simulink model "DCDC_SEPIC_TopLevelModel"  (R2023b)
settings: Solver=ode23t  StartTime=0.0  StopTime=10  FixedStep=ts500us  RelTol=1e-3
StartFcn:
  | try
  | resetTiLeds(objLEDs);
  | end
undefined symbols (not defined in the file): GPTRIP1SEL, GPTRIP2SEL, operatingMode, psu_V, timer_period_LED, timer_period_SEPIC, ts, ts100ms, ts10ms, ts1ms, ts500us, TZ1, TZ2
libraries: fl_lib x34, ee_lib x18, dspstat3 x17, SEPIC_utilities x16, c2802xlib x13, nesl_utility x10, simulink x4, batteryecm_lib x3
(part 1 of 2)
CloseFcn:
  | clear objLEDs; close all force; clc;
settings Model: ExtModeTrigDuration=8  Creator=vivekr  LastModifiedBy=vlenzi
settings SolverCC: AlgebraicLoopSolver=TrustRegion
settings DataIOCC: SaveFormat=StructureWithTime  SaveOutput=off  SaveTime=off  SignalLoggingName=logsOut
settings OptimizationCC: DefaultParameterBehavior=Inlined  UseDivisionForNetSlopeComputation=UseDivisionForReciprocalsOfIntegersOnly  EnhancedBackFolding=on  BooleansAsBitfields=on  PassReuseOutputArgsAs=Individual arguments  ExpressionDepthLimit=2147483647  StateBitsets=on  DataBitsets=on  ZeroExternalMemoryAtStartup=off  NoFixptDivByZeroProtection=on  EfficientFloat2IntCast=on  LifeSpan=1  MaxStackSize=64  SimCompilerOptimization=on  EfficientTunableParamExpr=on
settings DebuggingCC: ReadBeforeWriteMsg=DisableAll  WriteAfterWriteMsg=DisableAll  WriteAfterReadMsg=DisableAll  UnderspecifiedInitializationDetection=Classic  CheckExecutionContextPreStartOutputMsg=on  ParameterPrecisionLossMsg=none  FcnCallInpInsideContextMsg=warning  UnconnectedInputMsg=warning  UnconnectedOutputMsg=warning  UnconnectedLineMsg=warning  UniqueDataStoreMsg=error  AllowSymbolicDim=off  ModelReferenceSymbolNameMessage=none  StateNameClashWarn=warning  StrictBusMsg=ErrorOnBusTreatedAsVector  SymbolicDimsDataTypeCodeGenerationDiagnostic=none  SFUnexpectedBacktrackingDiag=warning  SFNoUnconditionalDefaultTransitionDiag=warning  SFExecutionAtInitializationDiag=none  ArithmeticOperatorsInVariantConditions=warning
settings HardwareCC: TargetHWDeviceType=Generic->32-bit Embedded Processor
settings ModelReferenceCC: EnableRefExpFcnMdlSchedulingChecks=on  CheckModelReferenceTargetMessage=none  PropagateSignalLabelsOutOfModel=off
settings SFSimCC: SimUseLocalCustomCode=off  MATLABDynamicMemAlloc=off
settings RTWCC: Description=Embedded Coder  SystemTargetFile=ert.tlc  TemplateMakefile=ert_default_tmf  GenerateReport=on  RTWVerbose=off  RTWUseLocalCustomCode=off  Toolchain=Texas Instruments Code Composer Studio (C2000)  IncludeHyperlinkInReport=on  CodeExecutionProfiling=on  CodeProfilingSaveOptions=AllData  CodeProfilingInstrumentation=coarse  GenerateTraceInfo=on  GenerateTraceReport=on  GenerateTraceReportSl=on  GenerateTraceReportSf=on  GenerateTraceReportEml=on  GenerateCodeMetricsReport=on  DLArmComputeVersion=19.05
settings CodeAppCC: ForceParamTrailComments=on  IgnoreCustomStorageClasses=off  SimulinkDataObjDesc=on  CustomSymbolStrGlobalVar=rt$N$M  CustomSymbolStrType=$N$M  CustomSymbolStrFcn=$N$M$F  CustomSymbolStrMacro=$N$M  InsertBlockDesc=on  StateflowObjectComments=on  InternalIdentifier=Classic
settings ERTTargetCC: UtilityFuncGeneration=Shared location  MultiwordLength=2048  IncludeMdlTerminateFcn=off  CombineSignalStateStructs=on  SupportNonFinite=off  SupportComplex=off  ExtModeStaticAllocSize=2048  ERTCustomFileTemplate=example_file_process.tlc  ERTFilePackagingFormat=CompactWithDataFile  ConvertIfToSwitch=off  SuppressUnreachableDefaultCases=off
settings ConfigComp: CovMetricSettings=dw  CovSaveCumulativeToWorkspaceVar=on  CovSaveSingleToWorkspaceVar=on  CovExternalEMLEnable=off  CovSFcnEnable=off
settings SimscapeCC: SimscapeUseOperatingPoints=on  SimscapeOperatingPoint=op_tm_average

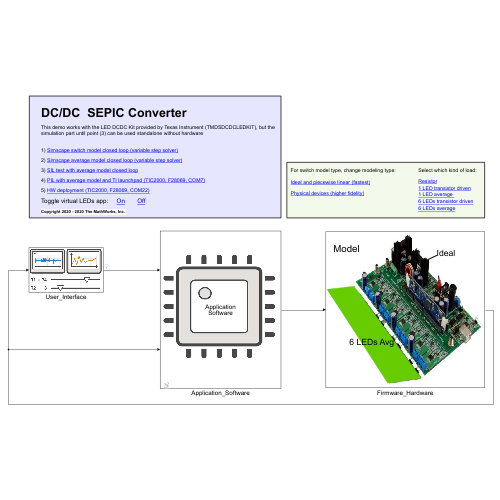
[thumbnail: Simulink's stored preview of the top-level diagram]
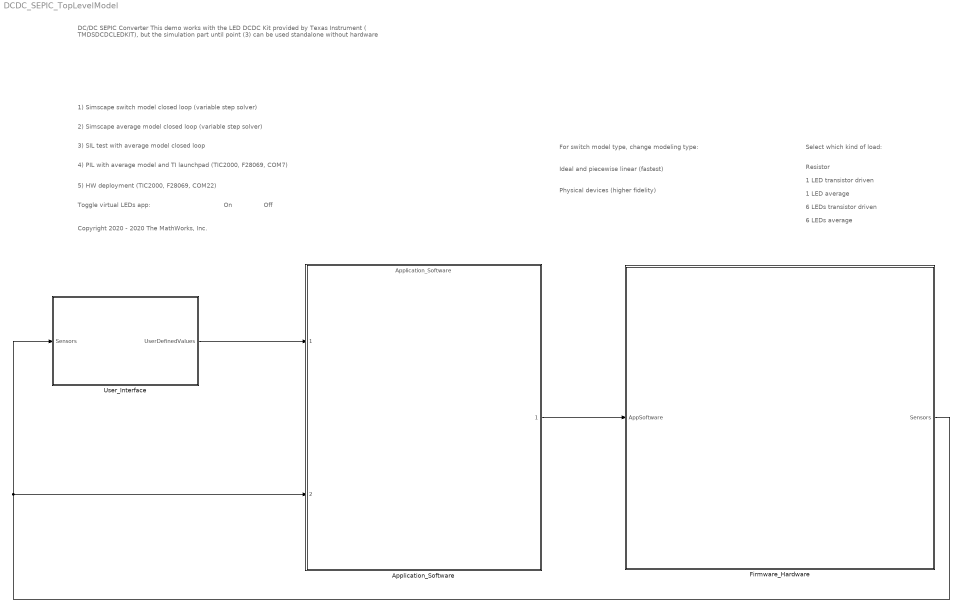
== system DCDC_SEPIC_TopLevelModel ==
  note: Copyright 2020 - 2020 The MathWorks, Inc.
  note: Ideal and piecewise linear (fastest)
  note: DC/DC SEPIC Converter
      |
      | This demo works with the LED DCDC Kit provided by Texas Instrument ( TMDSDCDCLEDKIT), but the simulation part until point (3) can be used standalone without hardware
  note: 5) HW deployment (TIC2000, F28069, COM22)
  note: 2) Simscape average model closed loop (variable step solver)
  note: 1) Simscape switch model closed loop (variable step solver)
  note: Physical devices (higher fidelity)
  note: For switch model type, change modeling type:
  note: 3) SIL test with average model closed loop
  note: Select which kind of load:
  note: Resistor
  note: 1 LED transistor driven
  note: 1 LED average
  note: 6 LEDs transistor driven
  note: 6 LEDs average
  note: Toggle virtual LEDs app:
  note: On
  note: Off
  note: 4) PIL with average model and TI launchpad (TIC2000, F28069, COM7)
  Application_Software : ModelReference  ModelNameDialog=Application_Software  SimulationMode=Normal  ModelReferenceVersion=1.589
      mask Display: image('cpu.png');disp('Application\nSoftware');
  Firmware_Hardware : Subsystem
      mask Display: image('SEPIC_converter_TI_Kit.jpg');text(0.05,0.9,'\fontsize{28}Model','texmode', 'on');plot([0.6 0.7],[0.8 0.85]);text(0.7,0.87,'\fontsize{25}Ideal','texmode', 'on');patch([0.39 0.01 0.18 0.6],[0.03 0.63 0.65 0.06], [0.4 0.8 0]);text(0.15,0.3,'\fontsize{25}6 LEDs Avg','texmode', 'on');
  User_Interface : Subsystem
      mask Display: image('user_interface.png');
  wires:
  User_Interface/1(UserDefinedValues) -> Application_Software/1
  Application_Software/1 -> Firmware_Hardware/1(AppSoftware)
  Firmware_Hardware/1(Sensors) -> User_Interface/1(Sensors), Application_Software/2

== system DCDC_SEPIC_TopLevelModel/Firmware_Hardware ==
  Bus Element In : Inport  PortName=AppSoftware  Element=dcpwmSEPIC
  Bus Element In1 : Inport  PortName=AppSoftware  Element=dcpwmLEDvector
  Hardware_Filter : Subsystem  Variant=on  VariantControl=Variant1  AllowZeroVariantControls=on
  Bus Element Out : Outport  PortName=Sensors  Element=voltSEPIC
  Bus Element Out1 : Outport  PortName=Sensors  Element=currSEPIC
  Bus Element Out2 : Outport  PortName=Sensors  Element=currLEDstrips
  Bus Element Out3 : Outport  PortName=Sensors  Element=voltPSU
  wires:
  Hardware_Filter/2(currSEPIC) -> Bus Element Out1/1  "currSEPIC"
  Hardware_Filter/3(currLEDstrips) -> Bus Element Out2/1  "currLEDstrips"
  Bus Element In1/1 -> Hardware_Filter/2(dcpwmLEDvector)
  Hardware_Filter/4(voltPSU) -> Bus Element Out3/1  "voltPSU"
  Hardware_Filter/1(voltSEPIC) -> Bus Element Out/1  "voltSEPIC"
  Bus Element In/1 -> Hardware_Filter/1(dcpwmSEPIC)

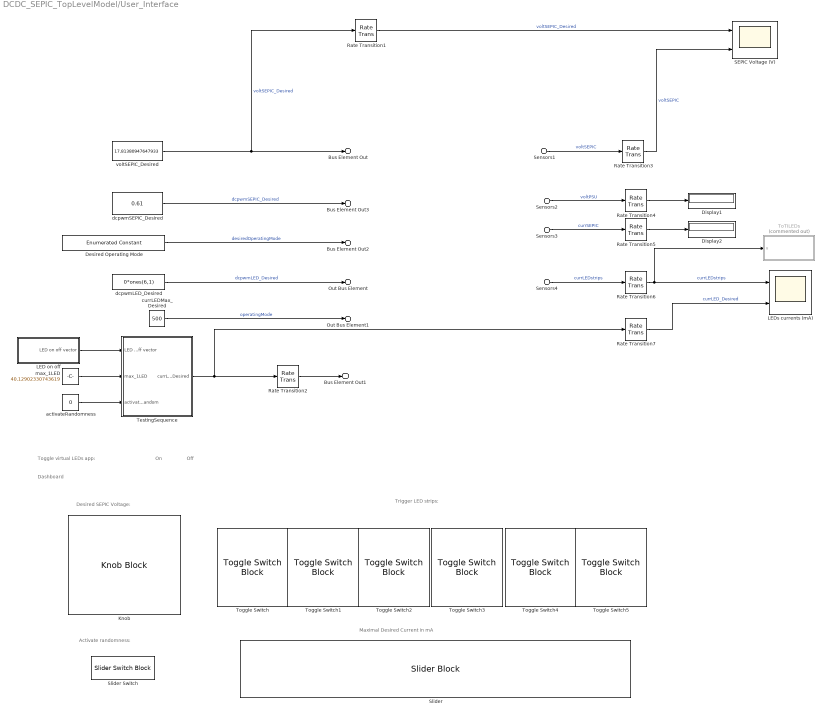
== system DCDC_SEPIC_TopLevelModel/User_Interface ==
  note: Maximal Desired Current in mA
  note: Dashboard
  note: Trigger LED strips:
  note: Desired SEPIC Voltage:
  note: Activate randomness:
  note: Toggle virtual LEDs app:
  note: On
  note: Off
  Sensors1 : Inport  PortName=Sensors  Element=voltSEPIC
  Sensors2 : Inport  PortName=Sensors  Element=voltPSU
  Sensors3 : Inport  PortName=Sensors  Element=currSEPIC
  Sensors4 : Inport  PortName=Sensors  Element=currLEDstrips
  Desired Operating Mode : simulink/Sources/Enumerated Constant  OutDataTypeStr=Enum: operatingMode  Value=operatingMode.AutomaticOperation  SampleTime=inf
  Display1 : Display
  Display2 : Display
  Knob : KnobBlock  LabelPosition=Hide  ScaleMin=9  ScaleMax=21  TickInterval=3
  LED on off : Subsystem
  LEDs currents (mA) : Scope  NumInputPorts=2
  Rate Transition{1,3..7} (6 alike) : RateTransition  Deterministic=off  OutPortSampleTime=ts10ms
  Rate Transition2 : RateTransition  Deterministic=off
  SEPIC Voltage (V) : Scope  NumInputPorts=2
  Slider : SliderBlock  LabelPosition=Hide  TickInterval=10
  Slider Switch : SliderSwitchBlock  LabelPosition=Hide
      settings: Values={{'Off', 'On'}, [0 1]}
  TestingSequence : Subsystem  Variant=on  VariantControlMode=label  VariantControl=Choice  LabelModeActiveChoice=Choice_1
  ToTILEDs : MATLAB Function  Commented=on  TreatAsAtomicUnit=on
  Toggle Switch{,1..5} (6 alike) : ToggleSwitchBlock  LabelPosition=Hide
      settings: Values={{'Off', 'On'}, [0 1]}
  activateRandomness : Constant  Value=0  OutDataTypeStr=single
  currLEDMax_Desired : Constant  Value=500  OutDataTypeStr=single
  dcpwmLED_Desired : Constant  Value=0*ones(6,1)  OutDataTypeStr=single
  dcpwmSEPIC_Desired : Constant  Value=0.61  OutDataTypeStr=single
  max_1LED : Constant  Value=40.12902330743619  OutDataTypeStr=single
  voltSEPIC_Desired : Constant  Value=17.81380947647933  OutDataTypeStr=single
  Bus Element Out : Outport  PortName=UserDefinedValues  Element=voltSEPIC_Desired
  Bus Element Out1 : Outport  PortName=UserDefinedValues  Element=currLED_Desired
  Bus Element Out2 : Outport  PortName=UserDefinedValues  Element=desiredOperatingMode
  Bus Element Out3 : Outport  PortName=UserDefinedValues  Element=dcpwmSEPIC_Desired
  Out Bus Element : Outport  PortName=UserDefinedValues  Element=dcpwmLED_Desired
  Out Bus Element1 : Outport  PortName=UserDefinedValues  Element=currLEDMax_Desired
  wires:
  voltSEPIC_Desired/1 -> Bus Element Out/1, Rate Transition1/1  "voltSEPIC_Desired"
  Desired Operating Mode/1 -> Bus Element Out2/1  "desiredOperatingMode"
  Sensors1/1 -> Rate Transition3/1  "voltSEPIC"
  Sensors2/1 -> Rate Transition4/1  "voltPSU"
  Sensors3/1 -> Rate Transition5/1  "currSEPIC"
  Sensors4/1 -> Rate Transition6/1  "currLEDstrips"
  dcpwmSEPIC_Desired/1 -> Bus Element Out3/1  "dcpwmSEPIC_Desired"
  dcpwmLED_Desired/1 -> Out Bus Element/1  "dcpwmLED_Desired"
  Rate Transition6/1 -> LEDs currents (mA)/1, ToTILEDs/1(u)  "currLEDstrips"
  currLEDMax_Desired/1 -> Out Bus Element1/1  "operatingMode"
  Rate Transition3/1 -> SEPIC Voltage (V)/2  "voltSEPIC"
  Rate Transition4/1 -> Display1/1
  Rate Transition5/1 -> Display2/1
  Rate Transition1/1 -> SEPIC Voltage (V)/1  "voltSEPIC_Desired"
  TestingSequence/1(currLED_Desired) -> Rate Transition2/1, Rate Transition7/1
  Rate Transition7/1 -> LEDs currents (mA)/2  "currLED_Desired"
  max_1LED/1 -> TestingSequence/2(max_1LED)
  LED on off/1(LED on off vector) -> TestingSequence/1(LED on off vector)
  activateRandomness/1 -> TestingSequence/3(activateRandom)
  Rate Transition2/1 -> Bus Element Out1/1

== system DCDC_SEPIC_TopLevelModel/Firmware_Hardware/Hardware_Filter ==
  dcpwmSEPIC : Inport  Unit=1
  dcpwmLEDvector : Inport  Port=2  Unit=1
  Simscape : Subsystem  VariantControl=Var_Plant==0
  TIC2000_F28069_Interfaces : Subsystem  VariantControl=Var_Plant==1
  voltSEPIC : Outport  Unit=V  VectorParamsAs1DForOutWhenUnconnected=off
  currSEPIC : Outport  Port=2  Unit=mA  VectorParamsAs1DForOutWhenUnconnected=off
  currLEDstrips : Outport  Port=3  Unit=mA  PortDimensions=6  VectorParamsAs1DForOutWhenUnconnected=off
  voltPSU : Outport  Port=4  Unit=V  VectorParamsAs1DForOutWhenUnconnected=off

== system DCDC_SEPIC_TopLevelModel/User_Interface/LED on off ==
  LED on off {1..4,6} (5 alike) : Constant  Value=0  OutDataTypeStr=single
  LED on off 5 : Constant  OutDataTypeStr=single
  Mux : Mux  Inputs=6
  LED on off vector : Outport
  wires:
  Mux/1 -> LED on off vector/1
  LED on off 6/1 -> Mux/6
  LED on off 2/1 -> Mux/2
  LED on off 4/1 -> Mux/4
  LED on off 1/1 -> Mux/1
  LED on off 5/1 -> Mux/5
  LED on off 3/1 -> Mux/3

== system DCDC_SEPIC_TopLevelModel/User_Interface/TestingSequence ==
  LED on off vector : Inport
  max_1LED : Inport  Port=2
  activateRandom : Inport  Port=3
  RandomPulses : Subsystem  VariantControl=Choice_1
  Vectorization : Subsystem  VariantControl=Choice
  currLED_Desired : Outport

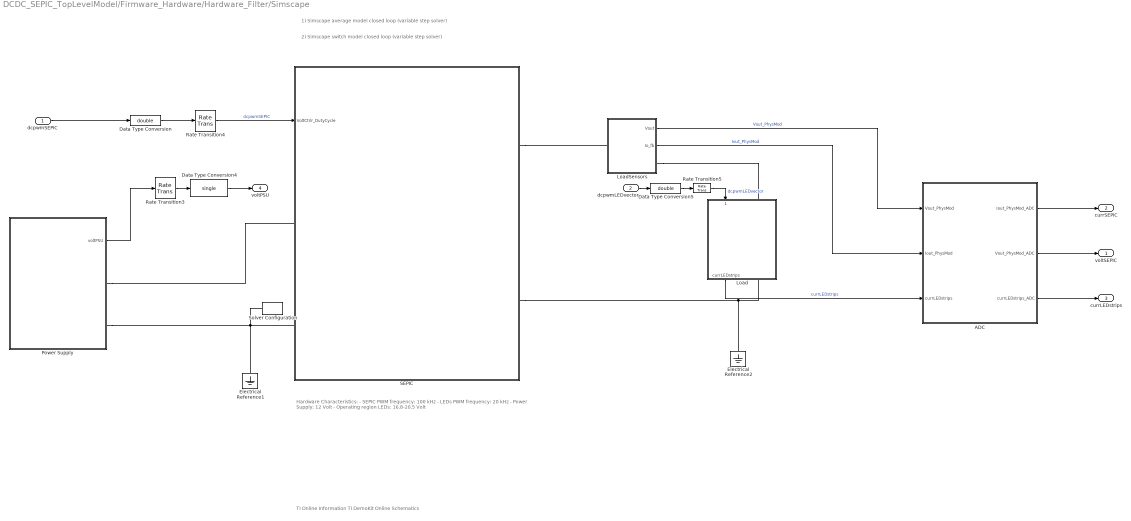
== system DCDC_SEPIC_TopLevelModel/Firmware_Hardware/Hardware_Filter/Simscape ==
  note: Hardware Characteristics:
      | - SEPIC PWM frequency: 100 kHz
      | - LEDs PWM frequency: 20 kHz
      | - Power Supply: 12 Volt
      | - Operating region LEDs: 16.8-20.5 Volt
  note: 2) Simscape switch model closed loop (variable step solver)
  note: 1) Simscape average model closed loop (variable step solver)
  note: TI Online Information
      | TI DemoKit Online Schematics
  dcpwmSEPIC : Inport  OutDataTypeStr=single  Unit=1  PortDimensions=1
  dcpwmLEDvector : Inport  Port=2  Unit=1
  ADC : Subsystem
      mask Display: disp('ADC');
  Data Type Conversion : DataTypeConversion  OutDataTypeStr=double  SaturateOnIntegerOverflow=off  RndMeth=Floor
  Data Type Conversion4 : DataTypeConversion  OutDataTypeStr=single  SaturateOnIntegerOverflow=off  RndMeth=Floor
  Data Type Conversion5 : DataTypeConversion  OutDataTypeStr=double  SaturateOnIntegerOverflow=off  RndMeth=Floor
  Electrical Reference1 : fl_lib/Electrical/Electrical Elements/Electrical Reference
  Electrical Reference2 : fl_lib/Electrical/Electrical Elements/Electrical Reference
  Load : Subsystem  Variant=on  VariantControlMode=label  VariantControl=Variant1  LabelModeActiveChoice=SixLEDStripsAvg
      mask Display: image('LED_Picture.jpg'); % Use "Edit Image" on toolstrip to change.
  LoadSensors : Subsystem
  Power Supply : Subsystem  Variant=on  VariantControlMode=label  VariantControl=Variant1  LabelModeActiveChoice=Battery
      mask Display:
      | % Plot points to set plot range
      | color('white');plot(1.5, 2.5);plot(-1.5, -2)
      | color('black');
      | % Battery icon
      | plot([0 0], [2.5 1.3])
      | plot([0 0], [-0.6 -1.6])
      | patch([-1 1 1 -1]*0.4, [1 1 -1 -1]*0.15+0.7,[0;0;0]);
      | patch([-1 1 1 -1]*0.4, [1 1 -1 -1]*0.15-0.6,[0;0;0]);
      | patch([-1 1 1 -1]*0.8, [1 1 -1 -1]*0.15+1.3,[0;0;0]);
      | patch([-1 1 1 -1]*0.8, [1 1 -1 -1]*0.15+0.0,[0;0;0]);
      | text(1.2, 0.25,'+');
      | text(1.2,-1.1,'_');
      | text(1.2,1.8,'m');
  Rate Transition3 : RateTransition  OutPortSampleTime=ts100ms
  Rate Transition4 : RateTransition
  Rate Transition5 : RateTransition
  SEPIC : Subsystem  Variant=on  VariantControl=Variant1
      mask Display: image('dc_dc_converter.png'); % Use "Edit Image" on toolstrip to change.
  Solver Configuration : nesl_utility/Solver Configuration  PhysicalDomain=network_engine_domain  SubClassName=solver  LeftPortType=input  RightPortType=generic  Tones=[]  Harmonics=[]  SimulateNoise=off  Profile=off  UseLocalSampling=off  EnableSwitchedLinearOptims=on  FrequencyDomain=off  UseCCode=off  RelTol=0.001  AbsTol=1e-06  MinStep=1e-09  ToWorkspace=off  RevertToSquareIcSolve=off  NumHomotopyIterations=100  PhasorMode=off  PhasorModeNumHarmonics=1  ConsistencySolver=NEWTON_FTOL  IndexReductionMethod=DerivativeReplacement  DoDC=off  ResidualTolerance=1e-9  ConsistencyTolSource=GLOBAL  ConsistencyAbsTol=0.001  ConsistencyRelTol=0.001  ConsistencyTolFactor=0.001  UseLocalSolver=off  LocalSolverChoice=NE_BACKWARD_EULER_ADVANCER  ResolveIndetEquations=on  FunctionEvalNumThread=1  LocalSolverSampleTime=2e-7  DoFixedCost=off  MaxNonlinIter=2  MaxModeIter=2  ComputeImpulses=off  ImpulseIterations=2  LinearAlgebra=Sparse  LinearAlgebraNumThread=0  EquationFormulation=NE_TIME_EF  DelaysMemoryBudget=1024  AutomaticFiltering=on  FilteringTimeConstant=0.001  PartitionStorageMethod=AS_NEEDED  PartitionMemoryBudget=1024  PartitionMethod=ROBUST  MultibodyUseLocalSolver=off  MultibodyLocalSolverChoice=ODE1  MultibodyLocalSolverSampleTime=0.001
  voltSEPIC : Outport  OutDataTypeStr=single  Unit=V  PortDimensions=1  VectorParamsAs1DForOutWhenUnconnected=off
  currSEPIC : Outport  Port=2  Unit=mA  VectorParamsAs1DForOutWhenUnconnected=off
  currLEDstrips : Outport  Port=3  Unit=mA  VectorParamsAs1DForOutWhenUnconnected=off
  voltPSU : Outport  Port=4  Unit=V  VectorParamsAs1DForOutWhenUnconnected=off
  wires:
  Data Type Conversion5/1 -> Rate Transition5/1
  dcpwmLEDvector/1 -> Data Type Conversion5/1
  dcpwmSEPIC/1 -> Data Type Conversion/1
  Rate Transition4/1 -> SEPIC/1(VoltCtrlr_DutyCycle)  "dcpwmSEPIC"
  Data Type Conversion/1 -> Rate Transition4/1
  Rate Transition5/1 -> Load/1(dcpwmLEDvector)  "dcpwmLEDvector"
  Rate Transition3/1 -> Data Type Conversion4/1
  Data Type Conversion4/1 -> voltPSU/1
  Power Supply/1(voltPSU) -> Rate Transition3/1
  LoadSensors/1(Vout) -> ADC/1(Vout_PhysMod)  "Vout_PhysMod"
  LoadSensors/2(Io_fb) -> ADC/2(Iout_PhysMod)  "Iout_PhysMod"
  Load/1(currLEDstrips) -> ADC/3(currLEDstrips)  "currLEDstrips"
  ADC/3(currLEDstrips_ADC) -> currLEDstrips/1
  ADC/2(Vout_PhysMod_ADC) -> voltSEPIC/1
  ADC/1(Iout_PhysMod_ADC) -> currSEPIC/1
  connections:
  LoadSensors/RConn1 -- Load/LConn1
  Electrical Reference2/LConn1 -- SEPIC/RConn2 -- Load/RConn1
  SEPIC/RConn1 -- LoadSensors/LConn1
  SEPIC/LConn2 -- Solver Configuration/RConn1 -- Electrical Reference1/LConn1 -- Power Supply/RConn2
  Power Supply/RConn1 -- SEPIC/LConn1

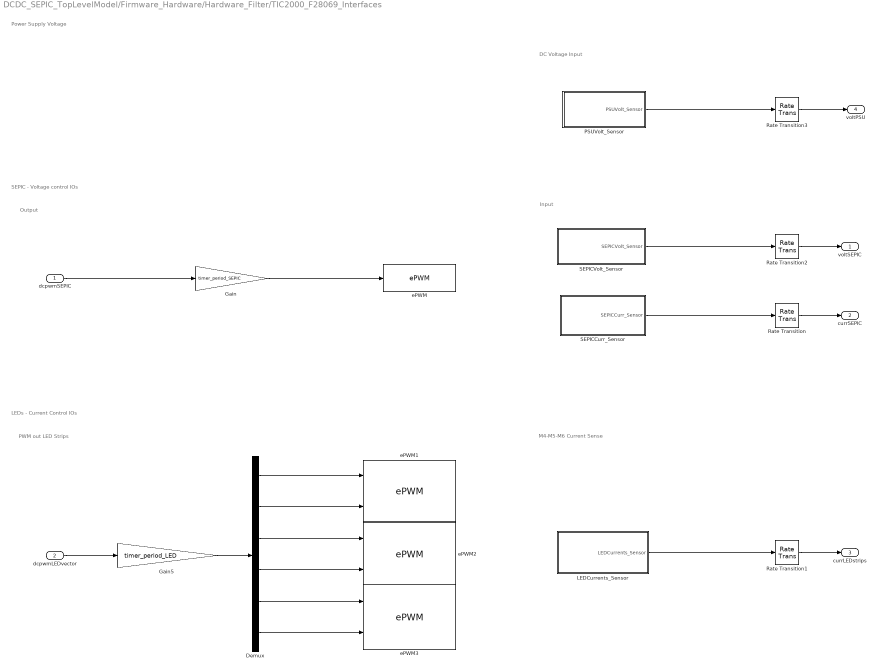
== system DCDC_SEPIC_TopLevelModel/Firmware_Hardware/Hardware_Filter/TIC2000_F28069_Interfaces ==
  note: Input
  note: SEPIC - Voltage control IOs
  note: Output
  note: PWM out LED Strips
  note: DC Voltage Input
  note: M4-M5-M6 Current Sense
  note: LEDs - Current Control IOs
  note: Power Supply Voltage
  dcpwmSEPIC : Inport  Unit=1
  dcpwmLEDvector : Inport  Port=2  Unit=1
  Demux : Demux  Outputs=6
  Gain : Gain  Gain=timer_period_SEPIC  OutMin=0  OutMax=70  OutDataTypeStr=int16  RndMeth=Simplest
  Gain5 : Gain  Gain=timer_period_LED  ParamDataTypeStr=int16  OutDataTypeStr=int16  RndMeth=Simplest
  LEDCurrents_Sensor : Subsystem  TreatAsAtomicUnit=on  SystemSampleTime=ts500us
  PSUVolt_Sensor : Subsystem  TreatAsAtomicUnit=on  SystemSampleTime=ts100ms
  Rate Transition{,1..3} (4 alike) : RateTransition  Deterministic=off
  SEPICCurr_Sensor : Subsystem  TreatAsAtomicUnit=on  SystemSampleTime=ts10ms
  SEPICVolt_Sensor : Subsystem  TreatAsAtomicUnit=on  SystemSampleTime=ts500us
  ePWM : c2802xlib/ePWM  PwmType=C2000  useModule=ePWM1  ePWMxLINKTBPRD=Not Linked  periodUnits=Clock cycles  timerSource=Specify via dialog  timerPeriod_clk=timer_period_SEPIC  timerPeriod_sec=0.00001  tbshadow=Immediate without using shadow  countingMode=Up  phaseActiveEnable=Disable  phaseDirection=Count down after sync  phaseActive=0  synchronizationEnable=off  dcaevt1Sync=off  dcbevt1Sync=off  synchronizationOption=Counter equals to zero (CTR=Zero)  perSynchronizationOption=Counter equals to period (CTR=PRD)  clockPrescale=1  HSclockPrescale=1  enswap=off  ePWMxAStatus=on  ePWMxAactionLogic1=Set  ePWMxAactionLogic2=Do nothing  ePWMxAactionLogic3=Clear  ePWMxAactionLogic4=Do nothing  ePWMxAactionLogic5=Do nothing  ePWMxAactionLogic6=Do nothing  ePWMxACSFenable=off  ePWMxACSFvalue=Forcing disable  ePWMxASFreload=Zero  ePWMxBStatus=off  ePWMxBactionLogic1=Do nothing  ePWMxBactionLogic2=Do nothing  ePWMxBactionLogic3=Do nothing  ePWMxBactionLogic4=Do nothing  ePWMxBactionLogic5=Do nothing  ePWMxBactionLogic6=Do nothing  ePWMxBCSFenable=off  ePWMxBCSFvalue=Forcing disable  ePWMxBSFreload=Zero  ePWNxBOutWay=off  ePWMxLINKCMPA=Not Linked  CMPAUnits=Clock cycles  CMPASource=Input port  CMPAValue_per=0  CMPAValue_clk=0  enCMPAshadow=Counter equals to period (CTR=PRD)  ePWMxLINKCMPB=Not Linked  CMPBUnits=Clock cycles  CMPBSource=Specify via dialog  CMPBValue_per=50  CMPBValue_clk=0  enCMPBshadow=Counter equals to zero (CTR=Zero)  ePWMxLINKCMPC=Not Linked  CMPCUnits=Clock cycles  CMPCSource=Specify via dialog  CMPCValue_per=50  CMPCValue_clk=32000  enCMPCshadow=Counter equals to zero (CTR=Zero)  ePWMxLINKCMPD=Not Linked  CMPDUnits=Clock cycles  CMPDSource=Specify via dialog  CMPDValue_per=50  CMPDValue_clk=32000  enCMPDshadow=Counter equals to zero (CTR=Zero)  enableDBePWMxA=off  enableDBePWMxB=off  enhalfcycle=off  DBpolarity=Active high (AH)  DBedgeDelay=Positive  DBSource_ePWMxA=ePWMxA  DBSource_ePWMxB=ePWMxA  DBPeriodUnits=Clock cycles  DBperiodSource=Specify via dialog  REDperiod=10  FEDperiod=10  REDperiod_sec=0  FEDperiod_sec=0  LoadModeDBRED=Immediate without using shadow  LoadModeDBFED=Immediate without using shadow  adcstartModuleA=on  adcrequestEventA=First event  adcstartEventA=Counter equals to zero (CTR=Zero)  adcstartEventA_type2=Digital Compare Module A Event 1 start of conversion (DCAEVT1.soc)  adcstartModuleB=off  adcrequestEventB=First event  adcstartEventB=Counter equals to zero (CTR=Zero)  adcstartEventB_type2=Counter equals to zero (CTR=Zero)  intEn=off  intPrd=First event  intSel=Counter equals to period (CTR=PRD)  intSel_type2=Counter equals to zero (CTR=Zero)  hrpe=off  enHRPWM=off  HRPWM_LoadMode=Counter equals to period (CTR=PRD)  HRPWM_CTLMode=Duty or Period control mode  HRPWM_EDGMode=Falling edge  hrpeb=off  enHRPWMB=off  HRPWM_LoadModeB=Counter equals to zero (CTR=ZERO)  HRPWM_CTLModeB=Duty or Period control mode  HRPWM_EDGModeB=Both edge  enHRDBRED=off  enHRDBFED=off  enSFO=off  enautoconv=off  chopperEnable=off  chopperFrequency=1  chopperFirstwidth=1  chopperDuty=12.5%  tripZonesource=Specify via dialog  tzselOSHT1=off  tzselOSHT2=off  tzselOSHT3=off  tzselOSHDCAEV1=off  tzselOSHDCBEV1=off  tzselCBC1=off  tzselCBC2=off  tzselCBC3=off  tzselCBCDCAEV2=off  tzselCBCDCBEV2=off  tzselOSHT4=off  tzselOSHT5=off  tzselOSHT6=off  tzselCBC4=off  tzselCBC5=off  tzselCBC6=off  enTzOstIntr=off  enTzCbcIntr=off  enTzDCAEVT1Intr=off  enTzDCAEVT2Intr=off  enTzDCBEVT1Intr=off  enTzDCBEVT2Intr=off  ePWMxAforced=No action  ePWMxBforced=No action  DCAEVT1forced=No action  DCBEVT1forced=No action  DCAEVT2forced=No action  DCBEVT2forced=No action  dcah=COMP1OUT input  dcal=Trip Zone 2 input (TZ2)  dcbh=Trip Zone 1 input (TZ1)  dcbl=Trip Zone 2 input (TZ2)  dcah_type2=GPTRIP1SEL/(TZ1)  dcal_type2=GPTRIP2SEL/(TZ2)  dcbh_type2=GPTRIP1SEL/(TZ1)  dcbl_type2=GPTRIP2SEL/(TZ2)  gendcaevt1=DCAH=high and DCAL=don't care  gendcaevt2=Event disabled  gendcbevt1=Event disabled  gendcbevt2=Event disabled  dcaevt1src=DCAEVT1 with async  dcaevt2src=DCAEVT2 with sync  dcbevt1src=DCBEVT1 with sync  dcbevt2src=DCBEVT2 with sync  pulsesel=Counter equals to zero (CTR=Zero)  blankinv=off  blankoffset=0  blankwidth=0  evsrcsel=Filtered version of DCAEVT1 (DCAEVT1FILT)  encape=off
  ePWM1 : c2802xlib/ePWM  PwmType=C2000  useModule=ePWM2  ePWMxLINKTBPRD=Not Linked  periodUnits=Clock cycles  timerSource=Specify via dialog  timerPeriod_clk=timer_period_LED  timerPeriod_sec=0.0001  tbshadow=Immediate without using shadow  countingMode=Up  phaseActiveEnable=Disable  phaseDirection=Count down after sync  phaseActive=timer_period_LED_phase1  synchronizationEnable=off  dcaevt1Sync=off  dcbevt1Sync=off  synchronizationOption=Counter equals to zero (CTR=Zero)  perSynchronizationOption=Counter equals to period (CTR=PRD)  clockPrescale=1  HSclockPrescale=1  enswap=off  ePWMxAStatus=on  ePWMxAactionLogic1=Set  ePWMxAactionLogic2=Do nothing  ePWMxAactionLogic3=Clear  ePWMxAactionLogic4=Do nothing  ePWMxAactionLogic5=Do nothing  ePWMxAactionLogic6=Do nothing  ePWMxACSFenable=off  ePWMxACSFvalue=Forcing disable  ePWMxASFreload=Zero  ePWMxBStatus=on  ePWMxBactionLogic1=Set  ePWMxBactionLogic2=Do nothing  ePWMxBactionLogic3=Do nothing  ePWMxBactionLogic4=Do nothing  ePWMxBactionLogic5=Clear  ePWMxBactionLogic6=Do nothing  ePWMxBCSFenable=off  ePWMxBCSFvalue=Forcing disable  ePWMxBSFreload=Zero  ePWNxBOutWay=off  ePWMxLINKCMPA=Not Linked  CMPAUnits=Clock cycles  CMPASource=Input port  CMPAValue_per=0  CMPAValue_clk=0  enCMPAshadow=Counter equals to period (CTR=PRD)  ePWMxLINKCMPB=Not Linked  CMPBUnits=Clock cycles  CMPBSource=Input port  CMPBValue_per=50  CMPBValue_clk=0  enCMPBshadow=Counter equals to period (CTR=PRD)  ePWMxLINKCMPC=Not Linked  CMPCUnits=Clock cycles  CMPCSource=Specify via dialog  CMPCValue_per=50  CMPCValue_clk=32000  enCMPCshadow=Counter equals to zero (CTR=Zero)  ePWMxLINKCMPD=Not Linked  CMPDUnits=Clock cycles  CMPDSource=Specify via dialog  CMPDValue_per=50  CMPDValue_clk=32000  enCMPDshadow=Counter equals to zero (CTR=Zero)  enableDBePWMxA=off  enableDBePWMxB=off  enhalfcycle=off  DBpolarity=Active high (AH)  DBedgeDelay=Positive  DBSource_ePWMxA=ePWMxA  DBSource_ePWMxB=ePWMxA  DBPeriodUnits=Clock cycles  DBperiodSource=Specify via dialog  REDperiod=10  FEDperiod=10  REDperiod_sec=0  FEDperiod_sec=0  LoadModeDBRED=Immediate without using shadow  LoadModeDBFED=Immediate without using shadow  adcstartModuleA=on  adcrequestEventA=First event  adcstartEventA=Counter equals to period (CTR=PRD)  adcstartEventA_type2=Digital Compare Module A Event 1 start of conversion (DCAEVT1.soc)  adcstartModuleB=on  adcrequestEventB=First event  adcstartEventB=Counter equals to period (CTR=PRD)  adcstartEventB_type2=Counter equals to zero (CTR=Zero)  intEn=off  intPrd=First event  intSel=Counter equals to period (CTR=PRD)  intSel_type2=Counter equals to zero (CTR=Zero)  hrpe=off  enHRPWM=off  HRPWM_LoadMode=Counter equals to period (CTR=PRD)  HRPWM_CTLMode=Duty or Period control mode  HRPWM_EDGMode=Falling edge  hrpeb=off  enHRPWMB=off  HRPWM_LoadModeB=Counter equals to zero (CTR=ZERO)  HRPWM_CTLModeB=Duty or Period control mode  HRPWM_EDGModeB=Both edge  enHRDBRED=off  enHRDBFED=off  enSFO=off  enautoconv=off  chopperEnable=off  chopperFrequency=1  chopperFirstwidth=1  chopperDuty=12.5%  tripZonesource=Specify via dialog  tzselOSHT1=off  tzselOSHT2=off  tzselOSHT3=off  tzselOSHDCAEV1=off  tzselOSHDCBEV1=off  tzselCBC1=off  tzselCBC2=off  tzselCBC3=off  tzselCBCDCAEV2=off  tzselCBCDCBEV2=off  tzselOSHT4=off  tzselOSHT5=off  tzselOSHT6=off  tzselCBC4=off  tzselCBC5=off  tzselCBC6=off  enTzOstIntr=off  enTzCbcIntr=off  enTzDCAEVT1Intr=off  enTzDCAEVT2Intr=off  enTzDCBEVT1Intr=off  enTzDCBEVT2Intr=off  ePWMxAforced=No action  ePWMxBforced=No action  DCAEVT1forced=No action  DCBEVT1forced=No action  DCAEVT2forced=No action  DCBEVT2forced=No action  dcah=COMP1OUT input  dcal=Trip Zone 2 input (TZ2)  dcbh=COMP1OUT input  dcbl=Trip Zone 2 input (TZ2)  dcah_type2=GPTRIP1SEL/(TZ1)  dcal_type2=GPTRIP2SEL/(TZ2)  dcbh_type2=GPTRIP1SEL/(TZ1)  dcbl_type2=GPTRIP2SEL/(TZ2)  gendcaevt1=DCAH=high and DCAL=don't care  gendcaevt2=Event disabled  gendcbevt1=Event disabled  gendcbevt2=Event disabled  dcaevt1src=DCAEVT1 with async  dcaevt2src=DCAEVT2 with sync  dcbevt1src=DCBEVT1 with sync  dcbevt2src=DCBEVT2 with sync  pulsesel=Counter equals to zero (CTR=Zero)  blankinv=off  blankoffset=0  blankwidth=0  evsrcsel=Filtered version of DCAEVT1 (DCAEVT1FILT)  encape=off
  ePWM2 : c2802xlib/ePWM  PwmType=C2000  useModule=ePWM3  ePWMxLINKTBPRD=Not Linked  periodUnits=Clock cycles  timerSource=Specify via dialog  timerPeriod_clk=timer_period_LED  timerPeriod_sec=0.0001  tbshadow=Immediate without using shadow  countingMode=Up  phaseActiveEnable=Set counter to phase value specified via dialog  phaseDirection=Count down after sync  phaseActive=timer_period_LED_phase2  synchronizationEnable=off  dcaevt1Sync=off  dcbevt1Sync=off  synchronizationOption=Counter equals to compare B (CTR=CMPB)  perSynchronizationOption=Counter equals to period (CTR=PRD)  clockPrescale=1  HSclockPrescale=1  enswap=off  ePWMxAStatus=on  ePWMxAactionLogic1=Set  ePWMxAactionLogic2=Do nothing  ePWMxAactionLogic3=Clear  ePWMxAactionLogic4=Do nothing  ePWMxAactionLogic5=Do nothing  ePWMxAactionLogic6=Do nothing  ePWMxACSFenable=off  ePWMxACSFvalue=Forcing disable  ePWMxASFreload=Zero  ePWMxBStatus=on  ePWMxBactionLogic1=Set  ePWMxBactionLogic2=Do nothing  ePWMxBactionLogic3=Do nothing  ePWMxBactionLogic4=Do nothing  ePWMxBactionLogic5=Clear  ePWMxBactionLogic6=Do nothing  ePWMxBCSFenable=off  ePWMxBCSFvalue=Forcing disable  ePWMxBSFreload=Zero  ePWNxBOutWay=off  ePWMxLINKCMPA=Not Linked  CMPAUnits=Clock cycles  CMPASource=Input port  CMPAValue_per=0  CMPAValue_clk=0  enCMPAshadow=Counter equals to period (CTR=PRD)  ePWMxLINKCMPB=Not Linked  CMPBUnits=Clock cycles  CMPBSource=Input port  CMPBValue_per=50  CMPBValue_clk=0  enCMPBshadow=Counter equals to period (CTR=PRD)  ePWMxLINKCMPC=Not Linked  CMPCUnits=Clock cycles  CMPCSource=Specify via dialog  CMPCValue_per=50  CMPCValue_clk=32000  enCMPCshadow=Counter equals to zero (CTR=Zero)  ePWMxLINKCMPD=Not Linked  CMPDUnits=Clock cycles  CMPDSource=Specify via dialog  CMPDValue_per=50  CMPDValue_clk=32000  enCMPDshadow=Counter equals to zero (CTR=Zero)  enableDBePWMxA=off  enableDBePWMxB=off  enhalfcycle=off  DBpolarity=Active high (AH)  DBedgeDelay=Positive  DBSource_ePWMxA=ePWMxA  DBSource_ePWMxB=ePWMxA  DBPeriodUnits=Clock cycles  DBperiodSource=Specify via dialog  REDperiod=10  FEDperiod=10  REDperiod_sec=0  FEDperiod_sec=0  LoadModeDBRED=Immediate without using shadow  LoadModeDBFED=Immediate without using shadow  adcstartModuleA=on  adcrequestEventA=First event  adcstartEventA=Counter equals to period (CTR=PRD)  adcstartEventA_type2=Digital Compare Module A Event 1 start of conversion (DCAEVT1.soc)  adcstartModuleB=on  adcrequestEventB=First event  adcstartEventB=Counter equals to period (CTR=PRD)  adcstartEventB_type2=Counter equals to zero (CTR=Zero)  intEn=off  intPrd=First event  intSel=Counter equals to period (CTR=PRD)  intSel_type2=Counter equals to zero (CTR=Zero)  hrpe=off  enHRPWM=off  HRPWM_LoadMode=Counter equals to period (CTR=PRD)  HRPWM_CTLMode=Duty or Period control mode  HRPWM_EDGMode=Falling edge  hrpeb=off  enHRPWMB=off  HRPWM_LoadModeB=Counter equals to zero (CTR=ZERO)  HRPWM_CTLModeB=Duty or Period control mode  HRPWM_EDGModeB=Both edge  enHRDBRED=off  enHRDBFED=off  enSFO=off  enautoconv=off  chopperEnable=off  chopperFrequency=1  chopperFirstwidth=1  chopperDuty=12.5%  tripZonesource=Specify via dialog  tzselOSHT1=off  tzselOSHT2=off  tzselOSHT3=off  tzselOSHDCAEV1=off  tzselOSHDCBEV1=off  tzselCBC1=off  tzselCBC2=off  tzselCBC3=off  tzselCBCDCAEV2=off  tzselCBCDCBEV2=off  tzselOSHT4=off  tzselOSHT5=off  tzselOSHT6=off  tzselCBC4=off  tzselCBC5=off  tzselCBC6=off  enTzOstIntr=off  enTzCbcIntr=off  enTzDCAEVT1Intr=off  enTzDCAEVT2Intr=off  enTzDCBEVT1Intr=off  enTzDCBEVT2Intr=off  ePWMxAforced=No action  ePWMxBforced=No action  DCAEVT1forced=No action  DCBEVT1forced=No action  DCAEVT2forced=No action  DCBEVT2forced=No action  dcah=COMP1OUT input  dcal=Trip Zone 2 input (TZ2)  dcbh=COMP1OUT input  dcbl=Trip Zone 2 input (TZ2)  dcah_type2=GPTRIP1SEL/(TZ1)  dcal_type2=GPTRIP2SEL/(TZ2)  dcbh_type2=GPTRIP1SEL/(TZ1)  dcbl_type2=GPTRIP2SEL/(TZ2)  gendcaevt1=DCAH=high and DCAL=don't care  gendcaevt2=Event disabled  gendcbevt1=Event disabled  gendcbevt2=Event disabled  dcaevt1src=DCAEVT1 with async  dcaevt2src=DCAEVT2 with sync  dcbevt1src=DCBEVT1 with sync  dcbevt2src=DCBEVT2 with sync  pulsesel=Counter equals to zero (CTR=Zero)  blankinv=off  blankoffset=0  blankwidth=0  evsrcsel=Filtered version of DCAEVT1 (DCAEVT1FILT)  encape=off
  ePWM3 : c2802xlib/ePWM  PwmType=C2000  useModule=ePWM4  ePWMxLINKTBPRD=Not Linked  periodUnits=Clock cycles  timerSource=Specify via dialog  timerPeriod_clk=timer_period_LED  timerPeriod_sec=0.0001  tbshadow=Immediate without using shadow  countingMode=Up  phaseActiveEnable=Set counter to phase value specified via dialog  phaseDirection=Count down after sync  phaseActive=timer_period_LED_phase3  synchronizationEnable=off  dcaevt1Sync=off  dcbevt1Sync=off  synchronizationOption=Counter equals to compare B (CTR=CMPB)  perSynchronizationOption=Counter equals to period (CTR=PRD)  clockPrescale=1  HSclockPrescale=1  enswap=off  ePWMxAStatus=on  ePWMxAactionLogic1=Set  ePWMxAactionLogic2=Do nothing  ePWMxAactionLogic3=Clear  ePWMxAactionLogic4=Do nothing  ePWMxAactionLogic5=Do nothing  ePWMxAactionLogic6=Do nothing  ePWMxACSFenable=off  ePWMxACSFvalue=Forcing disable  ePWMxASFreload=Zero  ePWMxBStatus=on  ePWMxBactionLogic1=Set  ePWMxBactionLogic2=Do nothing  ePWMxBactionLogic3=Do nothing  ePWMxBactionLogic4=Do nothing  ePWMxBactionLogic5=Clear  ePWMxBactionLogic6=Do nothing  ePWMxBCSFenable=off  ePWMxBCSFvalue=Forcing disable  ePWMxBSFreload=Zero  ePWNxBOutWay=off  ePWMxLINKCMPA=Not Linked  CMPAUnits=Clock cycles  CMPASource=Input port  CMPAValue_per=0  CMPAValue_clk=0  enCMPAshadow=Counter equals to period (CTR=PRD)  ePWMxLINKCMPB=Not Linked  CMPBUnits=Clock cycles  CMPBSource=Input port  CMPBValue_per=50  CMPBValue_clk=0  enCMPBshadow=Counter equals to period (CTR=PRD)  ePWMxLINKCMPC=Not Linked  CMPCUnits=Clock cycles  CMPCSource=Specify via dialog  CMPCValue_per=50  CMPCValue_clk=32000  enCMPCshadow=Counter equals to zero (CTR=Zero)  ePWMxLINKCMPD=Not Linked  CMPDUnits=Clock cycles  CMPDSource=Specify via dialog  CMPDValue_per=50  CMPDValue_clk=32000  enCMPDshadow=Counter equals to zero (CTR=Zero)  enableDBePWMxA=off  enableDBePWMxB=off  enhalfcycle=off  DBpolarity=Active high (AH)  DBedgeDelay=Positive  DBSource_ePWMxA=ePWMxA  DBSource_ePWMxB=ePWMxA  DBPeriodUnits=Clock cycles  DBperiodSource=Specify via dialog  REDperiod=10  FEDperiod=10  REDperiod_sec=0  FEDperiod_sec=0  LoadModeDBRED=Immediate without using shadow  LoadModeDBFED=Immediate without using shadow  adcstartModuleA=on  adcrequestEventA=First event  adcstartEventA=Counter equals to period (CTR=PRD)  adcstartEventA_type2=Digital Compare Module A Event 1 start of conversion (DCAEVT1.soc)  adcstartModuleB=on  adcrequestEventB=First event  adcstartEventB=Counter equals to period (CTR=PRD)  adcstartEventB_type2=Counter equals to zero (CTR=Zero)  intEn=off  intPrd=First event  intSel=Counter equals to period (CTR=PRD)  intSel_type2=Counter equals to zero (CTR=Zero)  hrpe=off  enHRPWM=off  HRPWM_LoadMode=Counter equals to period (CTR=PRD)  HRPWM_CTLMode=Duty or Period control mode  HRPWM_EDGMode=Falling edge  hrpeb=off  enHRPWMB=off  HRPWM_LoadModeB=Counter equals to zero (CTR=ZERO)  HRPWM_CTLModeB=Duty or Period control mode  HRPWM_EDGModeB=Both edge  enHRDBRED=off  enHRDBFED=off  enSFO=off  enautoconv=off  chopperEnable=off  chopperFrequency=1  chopperFirstwidth=1  chopperDuty=12.5%  tripZonesource=Specify via dialog  tzselOSHT1=off  tzselOSHT2=off  tzselOSHT3=off  tzselOSHDCAEV1=off  tzselOSHDCBEV1=off  tzselCBC1=off  tzselCBC2=off  tzselCBC3=off  tzselCBCDCAEV2=off  tzselCBCDCBEV2=off  tzselOSHT4=off  tzselOSHT5=off  tzselOSHT6=off  tzselCBC4=off  tzselCBC5=off  tzselCBC6=off  enTzOstIntr=off  enTzCbcIntr=off  enTzDCAEVT1Intr=off  enTzDCAEVT2Intr=off  enTzDCBEVT1Intr=off  enTzDCBEVT2Intr=off  ePWMxAforced=No action  ePWMxBforced=No action  DCAEVT1forced=No action  DCBEVT1forced=No action  DCAEVT2forced=No action  DCBEVT2forced=No action  dcah=COMP1OUT input  dcal=Trip Zone 2 input (TZ2)  dcbh=COMP1OUT input  dcbl=Trip Zone 2 input (TZ2)  dcah_type2=GPTRIP1SEL/(TZ1)  dcal_type2=GPTRIP2SEL/(TZ2)  dcbh_type2=GPTRIP1SEL/(TZ1)  dcbl_type2=GPTRIP2SEL/(TZ2)  gendcaevt1=DCAH=high and DCAL=don't care  gendcaevt2=Event disabled  gendcbevt1=Event disabled  gendcbevt2=Event disabled  dcaevt1src=DCAEVT1 with async  dcaevt2src=DCAEVT2 with sync  dcbevt1src=DCBEVT1 with sync  dcbevt2src=DCBEVT2 with sync  pulsesel=Counter equals to zero (CTR=Zero)  blankinv=off  blankoffset=0  blankwidth=0  evsrcsel=Filtered version of DCAEVT1 (DCAEVT1FILT)  encape=off
  voltSEPIC : Outport  Unit=V  VectorParamsAs1DForOutWhenUnconnected=off
  currSEPIC : Outport  Port=2  Unit=mA  VectorParamsAs1DForOutWhenUnconnected=off
  currLEDstrips : Outport  Port=3  OutDataTypeStr=single  Unit=mA  PortDimensions=6
  voltPSU : Outport  Port=4  Unit=V  VectorParamsAs1DForOutWhenUnconnected=off
  wires:
  Gain/1 -> ePWM/1
  Demux/1 -> ePWM1/1
  Demux/2 -> ePWM1/2
  Demux/3 -> ePWM2/1
  Gain5/1 -> Demux/1
  Demux/4 -> ePWM2/2
  Demux/5 -> ePWM3/1
  Demux/6 -> ePWM3/2
  SEPICCurr_Sensor/1(SEPICCurr_Sensor) -> Rate Transition/1
  dcpwmSEPIC/1 -> Gain/1
  dcpwmLEDvector/1 -> Gain5/1
  SEPICVolt_Sensor/1(SEPICVolt_Sensor) -> Rate Transition2/1
  LEDCurrents_Sensor/1(LEDCurrents_Sensor) -> Rate Transition1/1
  PSUVolt_Sensor/1(PSUVolt_Sensor) -> Rate Transition3/1
  Rate Transition/1 -> currSEPIC/1
  Rate Transition1/1 -> currLEDstrips/1
  Rate Transition2/1 -> voltSEPIC/1
  Rate Transition3/1 -> voltPSU/1

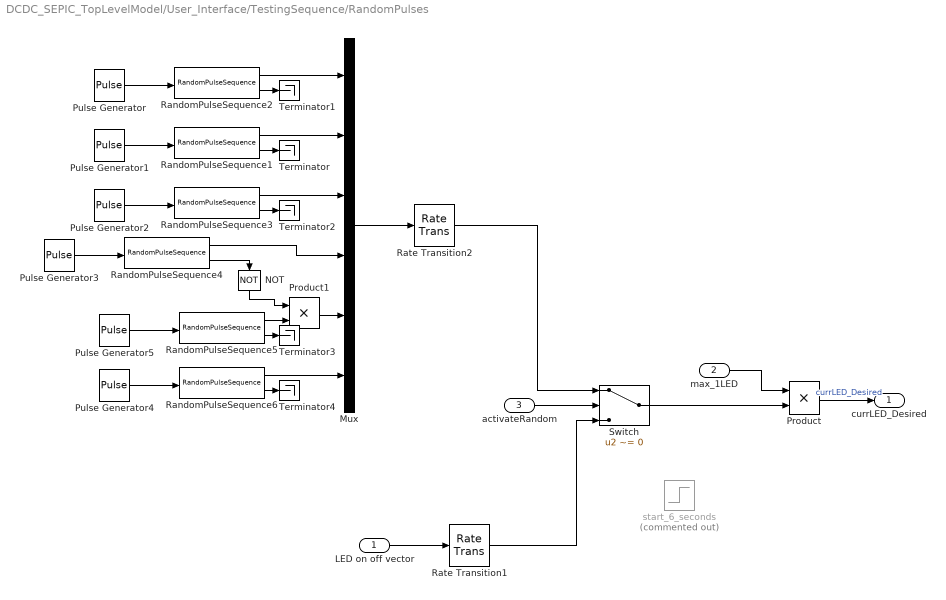
== system DCDC_SEPIC_TopLevelModel/User_Interface/TestingSequence/RandomPulses ==
  LED on off vector : Inport
  max_1LED : Inport  Port=2
  activateRandom : Inport  Port=3
  Mux : Mux  Inputs=6
  NOT : Logic  Operator=NOT  AllPortsSameDT=off  OutDataTypeStr=boolean
  Product : Product  OutDataTypeStr=single
  Product1 : Product
  Pulse Generator : DiscretePulseGenerator  Period=2*(1/ts500us)  PulseWidth=1*(1/ts500us)  SampleTime=ts500us
  Pulse Generator1 : DiscretePulseGenerator  Period=2*(1/ts500us)  PulseWidth=1*(1/ts500us)  PhaseDelay=1*400  SampleTime=ts500us
  Pulse Generator2 : DiscretePulseGenerator  Period=2*(1/ts500us)  PulseWidth=1*(1/ts500us)  PhaseDelay=2*400  SampleTime=ts500us
  Pulse Generator3 : DiscretePulseGenerator  Period=2*(1/ts500us)  PulseWidth=1*(1/ts500us)  PhaseDelay=3*400  SampleTime=ts500us
  Pulse Generator4 : DiscretePulseGenerator  Period=2*(1/ts500us)  PulseWidth=1*(1/ts500us)  PhaseDelay=5*400  SampleTime=ts500us
  Pulse Generator5 : DiscretePulseGenerator  Period=2*(1/ts500us)  PulseWidth=1*(1/ts500us)  PhaseDelay=4*400  SampleTime=ts500us
  RandomPulseSequence1 : SEPIC_utilities/RandomPulseSequence  seed=2  sampleTime=4
  RandomPulseSequence2 : SEPIC_utilities/RandomPulseSequence  seed=1  sampleTime=4
  RandomPulseSequence3 : SEPIC_utilities/RandomPulseSequence  seed=3  sampleTime=4
  RandomPulseSequence4 : SEPIC_utilities/RandomPulseSequence  seed=4  sampleTime=4
  RandomPulseSequence5 : SEPIC_utilities/RandomPulseSequence  seed=5  sampleTime=4
  RandomPulseSequence6 : SEPIC_utilities/RandomPulseSequence  seed=6  sampleTime=4
  Rate Transition1 : RateTransition  Deterministic=off
  Rate Transition2 : RateTransition  Deterministic=off
  Switch : Switch  Criteria=u2 ~= 0  SaturateOnIntegerOverflow=off  InputSameDT=off
  Terminator{,1..4} (5 alike) : Terminator
  start_6_seconds : Step  Commented=on  Time=6  SampleTime=ts1ms
  currLED_Desired : Outport
  wires:
  RandomPulseSequence5/2 -> Terminator3/1
  RandomPulseSequence6/2 -> Terminator4/1
  RandomPulseSequence6/1 -> Mux/6
  RandomPulseSequence2/2 -> Terminator1/1
  Pulse Generator3/1 -> RandomPulseSequence4/1
  Pulse Generator/1 -> RandomPulseSequence2/1
  RandomPulseSequence1/1 -> Mux/2
  Product1/1 -> Mux/5
  Pulse Generator2/1 -> RandomPulseSequence3/1
  RandomPulseSequence4/1 -> Mux/4
  RandomPulseSequence3/1 -> Mux/3
  RandomPulseSequence4/2 -> NOT/1
  RandomPulseSequence1/2 -> Terminator/1
  NOT/1 -> Product1/1
  Pulse Generator1/1 -> RandomPulseSequence1/1
  Pulse Generator5/1 -> RandomPulseSequence5/1
  Mux/1 -> Rate Transition2/1
  Pulse Generator4/1 -> RandomPulseSequence6/1
  RandomPulseSequence5/1 -> Product1/2
  RandomPulseSequence2/1 -> Mux/1
  RandomPulseSequence3/2 -> Terminator2/1
  Product/1 -> currLED_Desired/1  "currLED_Desired"
  max_1LED/1 -> Product/1
  activateRandom/1 -> Switch/2
  Switch/1 -> Product/2
  LED on off vector/1 -> Rate Transition1/1
  Rate Transition2/1 -> Switch/1
  Rate Transition1/1 -> Switch/3

== system DCDC_SEPIC_TopLevelModel/User_Interface/TestingSequence/Vectorization ==
  LED on off vector : Inport
  max_1LED : Inport  Port=2
  Product : Product  Inputs=3  OutDataTypeStr=single
  start_6_seconds : Step  Time=6  SampleTime=ts1ms
  currLED_Desired : Outport
  wires:
  start_6_seconds/1 -> Product/3
  Product/1 -> currLED_Desired/1  "currLED_Desired"
  max_1LED/1 -> Product/2
  LED on off vector/1 -> Product/1

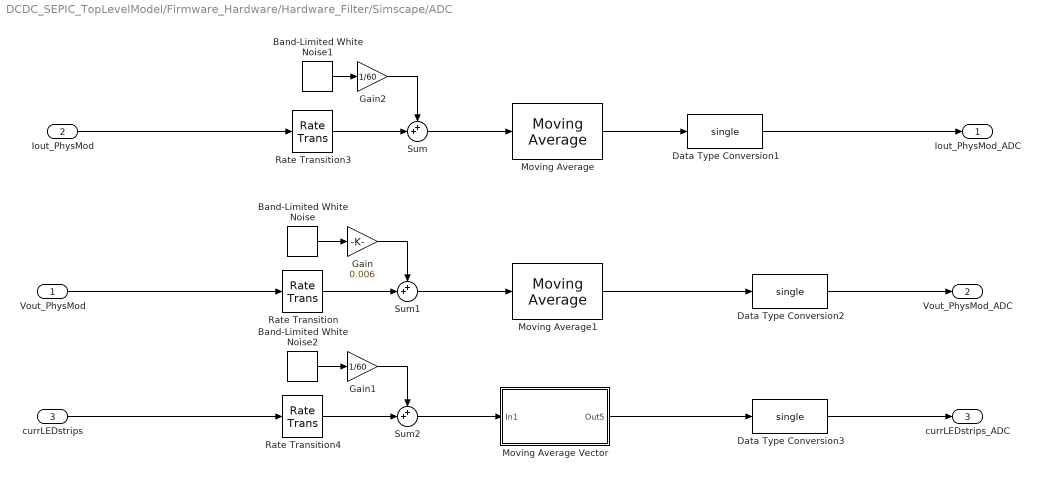
== system DCDC_SEPIC_TopLevelModel/Firmware_Hardware/Hardware_Filter/Simscape/ADC ==
  Vout_PhysMod : Inport
  Iout_PhysMod : Inport  Port=2
  currLEDstrips : Inport  Port=3
  Band-Limited White Noise : simulink/Sources/Band-Limited White Noise  Cov=0.1  Ts=ts500us  seed=[23341]
  Band-Limited White Noise1 : simulink/Sources/Band-Limited White Noise  Cov=2  Ts=ts10ms  seed=[23330]
  Band-Limited White Noise2 : simulink/Sources/Band-Limited White Noise  Cov=[2]  Ts=ts500us  seed=[23342]
  Data Type Conversion1 : DataTypeConversion  OutDataTypeStr=single  SaturateOnIntegerOverflow=off  RndMeth=Floor
  Data Type Conversion2 : DataTypeConversion  OutDataTypeStr=single  SaturateOnIntegerOverflow=off  RndMeth=Floor
  Data Type Conversion3 : DataTypeConversion  OutDataTypeStr=single  SaturateOnIntegerOverflow=off  RndMeth=Floor
  Gain : Gain  Gain=0.006
  Gain1 : Gain  Gain=1/60
  Gain2 : Gain  Gain=1/60
  Moving Average : dspstat3/Moving Average  Method=Exponential weighting  ForgettingFactorPort=off  SpecifyWindowLength=on  WindowLength=4  OverlapLength=3  AllowArbitraryInputLength=off  ForgettingFactor=0.93  SimulateUsing=Code generation
  Moving Average1 : dspstat3/Moving Average  Method=Exponential weighting  ForgettingFactorPort=off  SpecifyWindowLength=on  WindowLength=4  OverlapLength=3  AllowArbitraryInputLength=off  ForgettingFactor=0.93  SimulateUsing=Code generation
  Moving Average Vector : Subsystem
  Rate Transition : RateTransition  OutPortSampleTime=ts500us
  Rate Transition3 : RateTransition  OutPortSampleTime=ts10ms
  Rate Transition4 : RateTransition  OutPortSampleTime=ts500us
  Sum : Sum  Inputs=++|
  Sum1 : Sum  Inputs=++|
  Sum2 : Sum  Inputs=++|
  Iout_PhysMod_ADC : Outport
  Vout_PhysMod_ADC : Outport  Port=2
  currLEDstrips_ADC : Outport  Port=3
  wires:
  Vout_PhysMod/1 -> Rate Transition/1
  Data Type Conversion1/1 -> Iout_PhysMod_ADC/1
  Iout_PhysMod/1 -> Rate Transition3/1
  Moving Average/1 -> Data Type Conversion1/1
  currLEDstrips/1 -> Rate Transition4/1
  Data Type Conversion2/1 -> Vout_PhysMod_ADC/1
  Data Type Conversion3/1 -> currLEDstrips_ADC/1
  Rate Transition/1 -> Sum1/2
  Rate Transition3/1 -> Sum/2
  Rate Transition4/1 -> Sum2/2
  Band-Limited White Noise/1 -> Gain/1
  Band-Limited White Noise1/1 -> Gain2/1
  Band-Limited White Noise2/1 -> Gain1/1
  Sum/1 -> Moving Average/1
  Sum1/1 -> Moving Average1/1
  Moving Average1/1 -> Data Type Conversion2/1
  Gain/1 -> Sum1/1
  Gain1/1 -> Sum2/1
  Gain2/1 -> Sum/1
  Sum2/1 -> Moving Average Vector/1(In1)
  Moving Average Vector/1(Out5) -> Data Type Conversion3/1

== system DCDC_SEPIC_TopLevelModel/Firmware_Hardware/Hardware_Filter/Simscape/Load ==
  dcpwmLEDvector : Inport
  1 LED Strip : Subsystem  VariantControl=SingleLEDStrip
  6 LED Strips : Subsystem  VariantControl=SixLEDStrips
  6 LED Strips Avg : Subsystem  VariantControl=SixLEDStripsAvg
  LED Strip Avg : Subsystem  VariantControl=SingleLEDStripAvg
  Test Resistor : Subsystem  VariantControl=Resistor
  - : PMIOPort  Side=Right
  + : PMIOPort  Port=2  Side=Left
  currLEDstrips : Outport  Unit=mA  VectorParamsAs1DForOutWhenUnconnected=off

== system DCDC_SEPIC_TopLevelModel/Firmware_Hardware/Hardware_Filter/Simscape/LoadSensors ==
  Current Sensor2 : fl_lib/Electrical/Electrical Sensors/Current Sensor
  Electrical Reference2 : fl_lib/Electrical/Electrical Elements/Electrical Reference
  PS-Simulink Converter : nesl_utility/PS-Simulink Converter  PhysicalDomain=network_engine_domain  SubClassName=ps_output  LeftPortType=input  RightPortType=output  PseudoPeriodic=off  Frequencies=[]  VectorFormat=1-D array  Unit=V  AffineConversion=off
  PS-Simulink Converter1 : nesl_utility/PS-Simulink Converter  PhysicalDomain=network_engine_domain  SubClassName=ps_output  LeftPortType=input  RightPortType=output  PseudoPeriodic=off  Frequencies=[]  VectorFormat=1-D array  Unit=mA  AffineConversion=off
  Voltage Sensor : fl_lib/Electrical/Electrical Sensors/Voltage Sensor
  + : PMIOPort  Side=Left
  - : PMIOPort  Port=2  Side=Right
  Vout : Outport  VectorParamsAs1DForOutWhenUnconnected=off
  Io_fb : Outport  Port=2  VectorParamsAs1DForOutWhenUnconnected=off
  wires:
  PS-Simulink Converter1/1 -> Io_fb/1  "I_load"
  PS-Simulink Converter/1 -> Vout/1  "Vout"
  connections:
  Voltage Sensor/RConn1 -- PS-Simulink Converter/LConn1
  Voltage Sensor/RConn2 -- Electrical Reference2/LConn1
  Current Sensor2/LConn1 -- Voltage Sensor/LConn1 -- +/RConn1
  Current Sensor2/RConn1 -- PS-Simulink Converter1/LConn1
  -/RConn1 -- Current Sensor2/RConn2

== system DCDC_SEPIC_TopLevelModel/Firmware_Hardware/Hardware_Filter/Simscape/Power Supply ==
  Battery : Subsystem  VariantControl=Battery
      mask Display:
      | % Plot points to set plot range
      | color('white');plot(1.5, 2.5);plot(-1.5, -2)
      | color('black');
      | % Battery icon
      | plot([0 0], [2.5 1.3])
      | plot([0 0], [-0.6 -1.6])
      | patch([-1 1 1 -1]*0.4, [1 1 -1 -1]*0.15+0.7,[0;0;0]);
      | patch([-1 1 1 -1]*0.4, [1 1 -1 -1]*0.15-0.6,[0;0;0]);
      | patch([-1 1 1 -1]*0.8, [1 1 -1 -1]*0.15+1.3,[0;0;0]);
      | patch([-1 1 1 -1]*0.8, [1 1 -1 -1]*0.15+0.0,[0;0;0]);
      | text(1.2, 0.25,'+');
      | text(1.2,-1.1,'_');
      | text(1.2,1.8,'m');
  Power Supply : Subsystem  VariantControl=PowerSupply
  + : PMIOPort  Side=Right
  - : PMIOPort  Port=2  Side=Right
  voltPSU : Outport

== system DCDC_SEPIC_TopLevelModel/Firmware_Hardware/Hardware_Filter/Simscape/SEPIC ==
  VoltCtrlr_DutyCycle : Inport
  Average_SEPIC : Subsystem  VariantControl=Var_Converter==3  ReferencedSubsystem=Average_SEPIC
  Controlled_Converter : Subsystem  VariantControl=Var_Converter==0
  SEPIC_Circuit : Subsystem  VariantControl=Var_Converter==2  ReferencedSubsystem=SEPIC_Circuit
  SteadyState_Converter : Subsystem  VariantControl=Var_Converter==1
  1+ : PMIOPort  Side=Left
  1- : PMIOPort  Port=2  Side=Left
  2+ : PMIOPort  Port=3  Side=Right
  2- : PMIOPort  Port=4  Side=Right

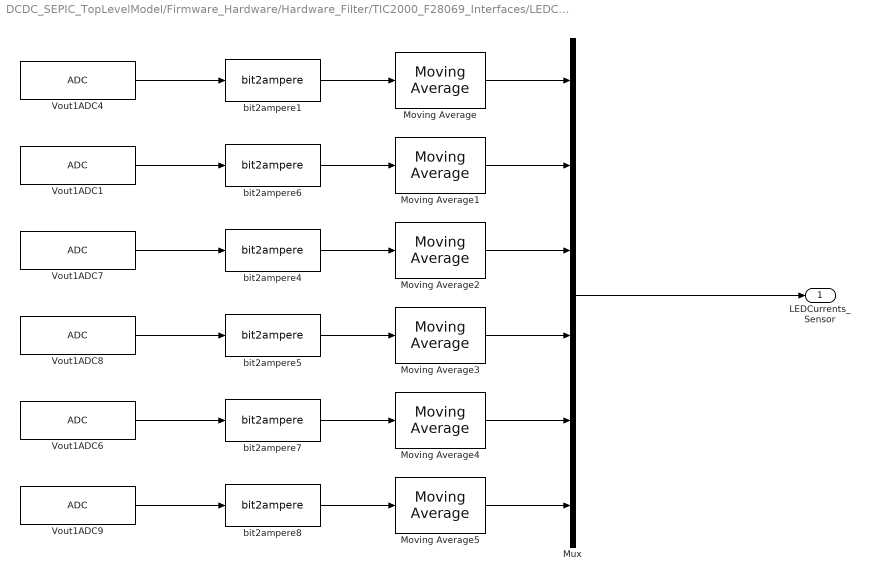
== system DCDC_SEPIC_TopLevelModel/Firmware_Hardware/Hardware_Filter/TIC2000_F28069_Interfaces/LEDCurrents_Sensor ==
  Moving Average{,1,3,5} (4 alike) : dspstat3/Moving Average  Method=Exponential weighting  ForgettingFactorPort=off  SpecifyWindowLength=on  WindowLength=4  ForgettingFactor=0.93  SimulateUsing=Code generation
  Moving Average2 : dspstat3/Moving Average  Method=Exponential weighting  ForgettingFactorPort=off  SpecifyWindowLength=on  WindowLength=4  ForgettingFactor=0.945  SimulateUsing=Code generation
  Moving Average4 : dspstat3/Moving Average  Method=Exponential weighting  ForgettingFactorPort=off  SpecifyWindowLength=on  WindowLength=4  ForgettingFactor=0.945  SimulateUsing=Code generation
  Mux : Mux  Inputs=6
  Vout1ADC1 : c2802xlib/ADC  blkParamProc=C2000  ADCModule=1  samplingMode=Single sample mode  ADCResolution=12-bit (Single-ended input)  useSOC1=SOC1  useSOC2=SOC0_SOC1  SOCAcquisitionWindow=7  SOCTriggerSource=ePWM2_ADCSOCB  SOCInterruptTrigger=No ADCINT  Ts=-1  dType=uint16  postInterrupt=off  interruptSel=ADCINT1  ADCINTContinuous=on  endma=off  chdma=1  conv1=ADCINA0  conv2=ADCINA0 and ADCINB0  conv1_Type4=ADCIN0  conv2_Type4=ADCIN0 and ADCIN1
  Vout1ADC4 : c2802xlib/ADC  blkParamProc=C2000  ADCModule=1  samplingMode=Single sample mode  ADCResolution=12-bit (Single-ended input)  useSOC1=SOC6  useSOC2=SOC0_SOC1  SOCAcquisitionWindow=7  SOCTriggerSource=ePWM2_ADCSOCA  SOCInterruptTrigger=No ADCINT  Ts=-1  dType=uint16  postInterrupt=off  interruptSel=ADCINT1  ADCINTContinuous=on  endma=off  chdma=1  conv1=ADCINB0  conv2=ADCINA0 and ADCINB0  conv1_Type4=ADCIN0  conv2_Type4=ADCIN0 and ADCIN1
  Vout1ADC6 : c2802xlib/ADC  blkParamProc=C2000  ADCModule=1  samplingMode=Single sample mode  ADCResolution=12-bit (Single-ended input)  useSOC1=SOC4  useSOC2=SOC0_SOC1  SOCAcquisitionWindow=7  SOCTriggerSource=ePWM4_ADCSOCA  SOCInterruptTrigger=No ADCINT  Ts=-1  dType=uint16  postInterrupt=off  interruptSel=ADCINT1  ADCINTContinuous=on  endma=off  chdma=1  conv1=ADCINB3  conv2=ADCINA0 and ADCINB0  conv1_Type4=ADCIN0  conv2_Type4=ADCIN0 and ADCIN1
  Vout1ADC7 : c2802xlib/ADC  blkParamProc=C2000  ADCModule=1  samplingMode=Single sample mode  ADCResolution=12-bit (Single-ended input)  useSOC1=SOC7  useSOC2=SOC0_SOC1  SOCAcquisitionWindow=7  SOCTriggerSource=ePWM3_ADCSOCA  SOCInterruptTrigger=No ADCINT  Ts=-1  dType=uint16  postInterrupt=off  interruptSel=ADCINT1  ADCINTContinuous=on  endma=off  chdma=1  conv1=ADCINB1  conv2=ADCINA0 and ADCINB0  conv1_Type4=ADCIN0  conv2_Type4=ADCIN0 and ADCIN1
  Vout1ADC8 : c2802xlib/ADC  blkParamProc=C2000  ADCModule=1  samplingMode=Single sample mode  ADCResolution=12-bit (Single-ended input)  useSOC1=SOC8  useSOC2=SOC0_SOC1  SOCAcquisitionWindow=7  SOCTriggerSource=ePWM3_ADCSOCB  SOCInterruptTrigger=No ADCINT  Ts=-1  dType=uint16  postInterrupt=off  interruptSel=ADCINT1  ADCINTContinuous=on  endma=off  chdma=1  conv1=ADCINB2  conv2=ADCINA0 and ADCINB0  conv1_Type4=ADCIN0  conv2_Type4=ADCIN0 and ADCIN1
  Vout1ADC9 : c2802xlib/ADC  blkParamProc=C2000  ADCModule=1  samplingMode=Single sample mode  ADCResolution=12-bit (Single-ended input)  useSOC1=SOC9  useSOC2=SOC0_SOC1  SOCAcquisitionWindow=7  SOCTriggerSource=ePWM4_ADCSOCB  SOCInterruptTrigger=No ADCINT  Ts=-1  dType=uint16  postInterrupt=off  interruptSel=ADCINT1  ADCINTContinuous=on  endma=off  chdma=1  conv1=ADCINA3  conv2=ADCINA0 and ADCINB0  conv1_Type4=ADCIN0  conv2_Type4=ADCIN0 and ADCIN1
  bit2ampere1 : SEPIC_utilities/bit2ampere  linear_coeff=Ifb_LED_LinearCoeff  offset=Ifb_LED_Offset1  zero_threshold=0
  bit2ampere4 : SEPIC_utilities/bit2ampere  linear_coeff=Ifb_LED_LinearCoeff  offset=Ifb_LED_Offset3  zero_threshold=5
  bit2ampere5 : SEPIC_utilities/bit2ampere  linear_coeff=Ifb_LED_LinearCoeff  offset=Ifb_LED_Offset4  zero_threshold=27
  bit2ampere6 : SEPIC_utilities/bit2ampere  linear_coeff=Ifb_LED_LinearCoeff  offset=Ifb_LED_Offset2  zero_threshold=0
  bit2ampere7 : SEPIC_utilities/bit2ampere  linear_coeff=Ifb_LED_LinearCoeff  offset=Ifb_LED_Offset5  zero_threshold=10
  bit2ampere8 : SEPIC_utilities/bit2ampere  linear_coeff=Ifb_LED_LinearCoeff  offset=Ifb_LED_Offset6  zero_threshold=10
  LEDCurrents_Sensor : Outport
  wires:
  Vout1ADC6/1 -> bit2ampere7/1
  Vout1ADC9/1 -> bit2ampere8/1
  Vout1ADC7/1 -> bit2ampere4/1
  Vout1ADC1/1 -> bit2ampere6/1
  Vout1ADC4/1 -> bit2ampere1/1
  Vout1ADC8/1 -> bit2ampere5/1
  Mux/1 -> LEDCurrents_Sensor/1
  bit2ampere1/1 -> Moving Average/1
  bit2ampere6/1 -> Moving Average1/1
  bit2ampere4/1 -> Moving Average2/1
  bit2ampere5/1 -> Moving Average3/1
  bit2ampere7/1 -> Moving Average4/1
  bit2ampere8/1 -> Moving Average5/1
  Moving Average5/1 -> Mux/6
  Moving Average4/1 -> Mux/5
  Moving Average2/1 -> Mux/3
  Moving Average1/1 -> Mux/2
  Moving Average3/1 -> Mux/4
  Moving Average/1 -> Mux/1
